simulink library "FixdToFloat"  (R2013b)
settings: Solver=ode45  StartTime=0.0  StopTime=10.0  RelTol=1e-3
settings Model: Creator=qzwc4r  LastModifiedBy=qzwc4r

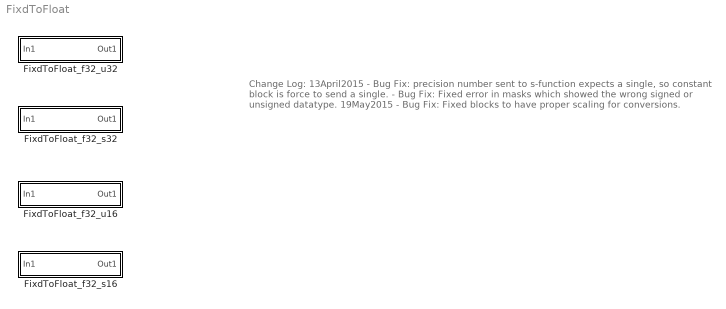
== system FixdToFloat ==
  note: Change Log:
      |
      | 13April2015
      | - Bug Fix: precision number sent to s-function expects a single, so constant block is force to send a single.
      | - Bug Fix: Fixed error in masks which showed the wrong signed or unsigned datatype.
      |
      | 19May2015
      | - Bug Fix: Fixed blocks to have proper scaling for conversions.
  FixdToFloat_f32_s16 : Subsystem  mask(FixdToFloat_f32_s16){Param1=0}
      mask prompts: Param1 "Precision"
      mask Display:
      | bits = 15;
      | pnum = Param1;
      | unum = bits-Param1;
      | 
      | port_label('output',1,'f32')
      | 
      | if pnum<0
      |    fptxt =  ['s' num2str(unum) 'pm' num2str(abs(pnum))];
      | elseif pnum>bits
      |    fptxt = ['sm' num2str(abs(unum)) 'p' num2str(pnum)];
      | else
      |    fptxt = ['s' num2str(unum) 'p' num2str(pnum)];
      | end
      | 
      | port_label('input',1,fptxt)
  FixdToFloat_f32_s32 : Subsystem  mask(FixdToFloat_f32_s32){Param1=0}
      mask prompts: Param1 "Precision"
      mask Display:
      | bits = 31;
      | pnum = Param1;
      | unum = bits-Param1;
      | 
      | port_label('output',1,'f32')
      | 
      | if pnum<0
      |    fptxt =  ['s' num2str(unum) 'pm' num2str(abs(pnum))];
      | elseif pnum>bits
      |    fptxt = ['sm' num2str(abs(unum)) 'p' num2str(pnum)];
      | else
      |    fptxt = ['s' num2str(unum) 'p' num2str(pnum)];
      | end
      | 
      | port_label('input',1,fptxt)
  FixdToFloat_f32_u16 : Subsystem  mask(FixdToFloat_f32_u16){Param1=0}
      mask prompts: Param1 "Precision"
      mask Display:
      | bits = 16;
      | pnum = Param1;
      | unum = bits-Param1;
      | 
      | port_label('output',1,'f32')
      | 
      | if pnum<0
      |    fptxt =  ['u' num2str(unum) 'pm' num2str(abs(pnum))];
      |    %fprintf(['u' num2str(unum) 'pm' num2str(abs(pnum))]);
      | elseif pnum>bits
      |    fptxt = ['um' num2str(abs(unum)) 'p' num2str(pnum)];
      |    %fprintf(['um' num2str(abs(unum)) 'p' num2str(pnum)]);
      | else
      |    fptxt = ['u' num2str(unum) 'p' num2str(pnum)];
      |    %fprintf(['u' num2str(unum) 'p' num2str(pnum)]);
      | end
      | 
      | port_label('input',1,fptxt)
  FixdToFloat_f32_u32 : Subsystem  mask(FixdToFloat_f32_u32){Param1=0}
      mask prompts: Param1 "Precision"
      mask Display:
      | bits = 32;
      | pnum = Param1;
      | unum = bits-Param1;
      | 
      | port_label('output',1,'f32')
      | 
      | if pnum<0
      |    fptxt =  ['u' num2str(unum) 'pm' num2str(abs(pnum))];
      |    %fprintf(['u' num2str(unum) 'pm' num2str(abs(pnum))]);
      | elseif pnum>bits
      |    fptxt = ['um' num2str(abs(unum)) 'p' num2str(pnum)];
      |    %fprintf(['um' num2str(abs(unum)) 'p' num2str(pnum)]);
      | else
      |    fptxt = ['u' num2str(unum) 'p' num2str(pnum)];
      |    %fprintf(['u' num2str(unum) 'p' num2str(pnum)]);
      | end
      | 
      | port_label('input',1,fptxt)

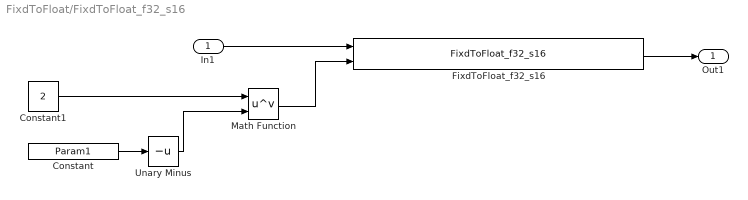
== system FixdToFloat/FixdToFloat_f32_s16 ==
  In1 : Inport
  Constant : Constant  Value=Param1  OutDataTypeStr=single
  Constant1 : Constant  Value=2  OutDataTypeStr=single
  FixdToFloat_f32_s16 : S-Function  FunctionName=FixdToFloat_f32_s16  EnableBusSupport=off  mask(Legacy Function){SFunctionSpec=single y1 = FixdToFloat_f32_s16( int16 u1, single u2), ShowSpec=on}
      mask prompts: ShowSpec "Display function specification"
      mask help:
      | This block allows you to call the legacy functions specified by the following Legacy Code Tool definition:
      | def.SFunctionName = 'FixdToFloat_f32_s16';
      | def.OutputFcnSpec = 'single y1 = FixdToFloat_f32_s16( int16 u1, single u2)';
      | def.HeaderFiles = {'NxtrFixdPt.h', 'Std_Types.h', 'Platform_Types.h', 'Compiler.h', 'Compiler_Cfg.h'};
      | def.IncPaths = {'..\SrcFiles'};
      mask Help: <p>This block was generated automatically by the Legacy Code Tool. For detailed help on this tool, call<a href="matlab:legacy_code('help')"> legacy_code('help')</a>.</p>
      mask Callback ShowSpec:
      | if strcmp(get_param(gcbh, 'ShowSpec'), 'on')
      |   set_param(gcbh, 'MaskDisplay', sprintf('fprintf(''%s'');', get_param(gcbh, 'SFunctionSpec')));
      | else
      |   set_param(gcbh, 'MaskDisplay', sprintf('fprintf(''%s'');', get_param(gcbh, 'FunctionName')));
      | end
      mask Display: fprintf('%s','single y1 = FixdToFloat_f32_s16( int16 u1, single u2)');
  Math Function : Math  Operator=pow  SaturateOnIntegerOverflow=on
  Unary Minus : UnaryMinus
  Out1 : Outport
  wires:
  FixdToFloat_f32_s16/1 -> Out1/1
  In1/1 -> FixdToFloat_f32_s16/1
  Math Function/1 -> FixdToFloat_f32_s16/2
  Constant1/1 -> Math Function/1
  Constant/1 -> Unary Minus/1
  Unary Minus/1 -> Math Function/2

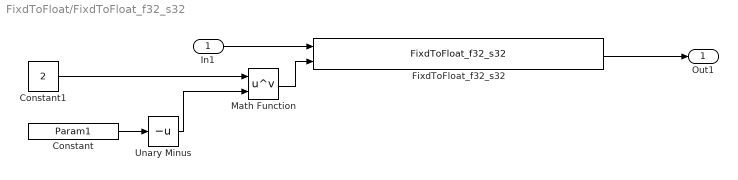
== system FixdToFloat/FixdToFloat_f32_s32 ==
  In1 : Inport
  Constant : Constant  Value=Param1  OutDataTypeStr=single
  Constant1 : Constant  Value=2  OutDataTypeStr=single
  FixdToFloat_f32_s32 : S-Function  FunctionName=FixdToFloat_f32_s32  EnableBusSupport=off  mask(Legacy Function){SFunctionSpec=single y1 = FixdToFloat_f32_s32( int32 u1, single u2), ShowSpec=on}
      mask prompts: ShowSpec "Display function specification"
      mask help:
      | This block allows you to call the legacy functions specified by the following Legacy Code Tool definition:
      | def.SFunctionName = 'FixdToFloat_f32_s32';
      | def.OutputFcnSpec = 'single y1 = FixdToFloat_f32_s32( int32 u1, single u2)';
      | def.HeaderFiles = {'NxtrFixdPt.h', 'Std_Types.h', 'Platform_Types.h', 'Compiler.h', 'Compiler_Cfg.h'};
      | def.IncPaths = {'..\SrcFiles'};
      mask Help: <p>This block was generated automatically by the Legacy Code Tool. For detailed help on this tool, call<a href="matlab:legacy_code('help')"> legacy_code('help')</a>.</p>
      mask Callback ShowSpec:
      | if strcmp(get_param(gcbh, 'ShowSpec'), 'on')
      |   set_param(gcbh, 'MaskDisplay', sprintf('fprintf(''%s'');', get_param(gcbh, 'SFunctionSpec')));
      | else
      |   set_param(gcbh, 'MaskDisplay', sprintf('fprintf(''%s'');', get_param(gcbh, 'FunctionName')));
      | end
      mask Display: fprintf('%s','single y1 = FixdToFloat_f32_s32( int32 u1, single u2)');
  Math Function : Math  Operator=pow  SaturateOnIntegerOverflow=on
  Unary Minus : UnaryMinus
  Out1 : Outport
  wires:
  FixdToFloat_f32_s32/1 -> Out1/1
  In1/1 -> FixdToFloat_f32_s32/1
  Math Function/1 -> FixdToFloat_f32_s32/2
  Constant1/1 -> Math Function/1
  Constant/1 -> Unary Minus/1
  Unary Minus/1 -> Math Function/2

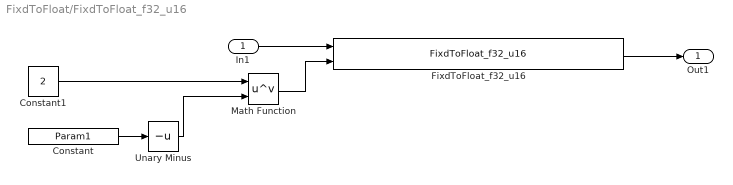
== system FixdToFloat/FixdToFloat_f32_u16 ==
  In1 : Inport
  Constant : Constant  Value=Param1  OutDataTypeStr=single
  Constant1 : Constant  Value=2  OutDataTypeStr=single
  FixdToFloat_f32_u16 : S-Function  FunctionName=FixdToFloat_f32_u16  EnableBusSupport=off  mask(Legacy Function){SFunctionSpec=single y1 = FixdToFloat_f32_u16(uint16 u1, single u2), ShowSpec=on}
      mask prompts: ShowSpec "Display function specification"
      mask help:
      | This block allows you to call the legacy functions specified by the following Legacy Code Tool definition:
      | def.SFunctionName = 'FixdToFloat_f32_u16';
      | def.OutputFcnSpec = 'single y1 = FixdToFloat_f32_u16(uint16 u1, single u2)';
      | def.HeaderFiles = {'NxtrFixdPt.h', 'Std_Types.h', 'Platform_Types.h', 'Compiler.h', 'Compiler_Cfg.h'};
      | def.IncPaths = {'..\SrcFiles'};
      mask Help: <p>This block was generated automatically by the Legacy Code Tool. For detailed help on this tool, call<a href="matlab:legacy_code('help')"> legacy_code('help')</a>.</p>
      mask Callback ShowSpec:
      | if strcmp(get_param(gcbh, 'ShowSpec'), 'on')
      |   set_param(gcbh, 'MaskDisplay', sprintf('fprintf(''%s'');', get_param(gcbh, 'SFunctionSpec')));
      | else
      |   set_param(gcbh, 'MaskDisplay', sprintf('fprintf(''%s'');', get_param(gcbh, 'FunctionName')));
      | end
      mask Display: fprintf('%s','single y1 = FixdToFloat_f32_u16(uint16 u1, single u2)');
  Math Function : Math  Operator=pow  SaturateOnIntegerOverflow=on
  Unary Minus : UnaryMinus
  Out1 : Outport
  wires:
  FixdToFloat_f32_u16/1 -> Out1/1
  In1/1 -> FixdToFloat_f32_u16/1
  Math Function/1 -> FixdToFloat_f32_u16/2
  Constant1/1 -> Math Function/1
  Constant/1 -> Unary Minus/1
  Unary Minus/1 -> Math Function/2

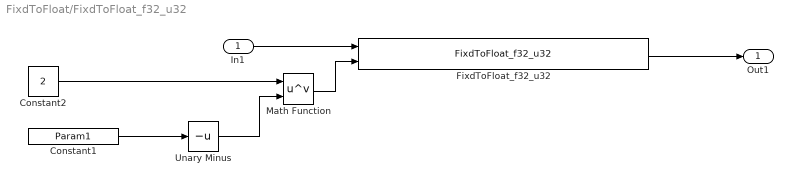
== system FixdToFloat/FixdToFloat_f32_u32 ==
  In1 : Inport
  Constant1 : Constant  Value=Param1  OutDataTypeStr=single
  Constant2 : Constant  Value=2  OutDataTypeStr=single
  FixdToFloat_f32_u32 : S-Function  FunctionName=FixdToFloat_f32_u32  EnableBusSupport=off  mask(Legacy Function){SFunctionSpec=single y1 = FixdToFloat_f32_u32(uint32 u1, single u2), ShowSpec=on}
      mask prompts: ShowSpec "Display function specification"
      mask help:
      | This block allows you to call the legacy functions specified by the following Legacy Code Tool definition:
      | def.SFunctionName = 'FixdToFloat_f32_u32';
      | def.OutputFcnSpec = 'single y1 = FixdToFloat_f32_u32(uint32 u1, single u2)';
      | def.HeaderFiles = {'NxtrFixdPt.h', 'Std_Types.h', 'Platform_Types.h', 'Compiler.h', 'Compiler_Cfg.h'};
      | def.IncPaths = {'..\SrcFiles'};
      mask Help: <p>This block was generated automatically by the Legacy Code Tool. For detailed help on this tool, call<a href="matlab:legacy_code('help')"> legacy_code('help')</a>.</p>
      mask Callback ShowSpec:
      | if strcmp(get_param(gcbh, 'ShowSpec'), 'on')
      |   set_param(gcbh, 'MaskDisplay', sprintf('fprintf(''%s'');', get_param(gcbh, 'SFunctionSpec')));
      | else
      |   set_param(gcbh, 'MaskDisplay', sprintf('fprintf(''%s'');', get_param(gcbh, 'FunctionName')));
      | end
      mask Display: fprintf('%s','single y1 = FixdToFloat_f32_u32(uint32 u1, single u2)');
  Math Function : Math  Operator=pow  SaturateOnIntegerOverflow=on
  Unary Minus : UnaryMinus
  Out1 : Outport
  wires:
  In1/1 -> FixdToFloat_f32_u32/1
  FixdToFloat_f32_u32/1 -> Out1/1
  Math Function/1 -> FixdToFloat_f32_u32/2
  Constant2/1 -> Math Function/1
  Constant1/1 -> Unary Minus/1
  Unary Minus/1 -> Math Function/2
